simulink model "arduino_stepper"  (R2014a)
settings: Solver=FixedStepDiscrete  SolverMode=SingleTasking  StartTime=0.0  StopTime=inf  FixedStep=0.010  RelTol=1e-3
libraries: arduinolib x5
settings Model: SimulationMode=external  ExtModeTrigDuration=2  Creator=hbosch  LastModifiedBy=hbosch
settings DataIOCC: LimitDataPoints=off  SaveOutput=off  SignalLogging=off  DSMLogging=off  SaveTime=off
settings OptimizationCC: InlineParams=on  StateBitsets=on  DataBitsets=on  OptimizeModelRefInitCode=on  LifeSpan=1
settings DebuggingCC: SignalInfNanChecking=error  SignalRangeChecking=error  ReadBeforeWriteMsg=EnableAllAsError  WriteAfterWriteMsg=EnableAllAsError  WriteAfterReadMsg=EnableAllAsError  AlgebraicLoopMsg=error  ArtificialAlgebraicLoopMsg=error  SaveWithDisabledLinksMsg=error  SaveWithParameterizedLinksMsg=error  UnderspecifiedInitializationDetection=Classic  MergeDetectMultiDrivingBlocksExec=error  CheckExecutionContextPreStartOutputMsg=on  CheckExecutionContextRuntimeOutputMsg=on  BlockPriorityViolationMsg=error  TimeAdjustmentMsg=warning  SolverPrmCheckMsg=none  InheritedTsInSrcMsg=error  DiscreteInheritContinuousMsg=error  SigSpecEnsureSampleTimeMsg=error  CheckMatrixSingularityMsg=error  IntegerOverflowMsg=error  ParameterUnderflowMsg=error  ParameterPrecisionLossMsg=error  ParameterTunabilityLossMsg=error  UnderSpecifiedDataTypeMsg=error  UnnecessaryDatatypeConvMsg=warning  VectorMatrixConversionMsg=error  SignalLabelMismatchMsg=error  UnconnectedInputMsg=error  UnconnectedOutputMsg=error  UnconnectedLineMsg=error  SFcnCompatibilityMsg=error  UniqueDataStoreMsg=error  BusObjectLabelMismatch=error  RootOutportRequireBusObject=error  AssertControl=DisableAll  ModelReferenceIOMsg=error  ModelReferenceIOMismatchMessage=error  ModelReferenceCSMismatchMessage=error  UnknownTsInhSupMsg=error  ModelReferenceDataLoggingMessage=error  StateNameClashWarn=warning
settings HardwareCC: ProdBitPerInt=16  ProdBitPerPointer=8  ProdIntDivRoundTo=Zero  ProdEndianess=LittleEndian  ProdWordSize=8  ProdHWDeviceType=Atmel->AVR
settings RTWCC: SystemTargetFile=realtime.tlc  GenerateMakefile=off  TemplateMakefile=realtime.tmf  Description=Run on Target Hardware  RTWVerbose=off  ProcessScript=realtime_make_rtw_hook
settings CodeAppCC: MangleLength=10
settings STFCustomTargetCC: TargetLibSuffix=.a  GenerateSampleERTMain=on  ConcurrentExecutionCompliant=off  GeneratePreprocessorConditionals=Use local settings  ERTCustomFileBanners=on  SupportNonInlinedSFcns=off  SupportVariableSizeSignals=on  MATLABClassNameForMDSCustomization=Simulink.SoftwareTarget.ERTCustomization  GRTInterface=off  SystemTargetFile=realtime.tlc
settings ERTTargetCC: CombineOutputUpdateFcns=off  SupportContinuousTime=on  SupportVariableSizeSignals=on  ExtModeTransport=3  ExtModeMexFile=ext_serial_win32_comm  ExtModeMexArgs=0 1 9600  ERTSrcFileBannerTemplate=realtime_code_template.cgt  ERTHdrFileBannerTemplate=realtime_code_template.cgt  ERTDataSrcFileTemplate=realtime_code_template.cgt  ERTDataHdrFileTemplate=realtime_code_template.cgt  ERTCustomFileTemplate=realtime_file_process.tlc

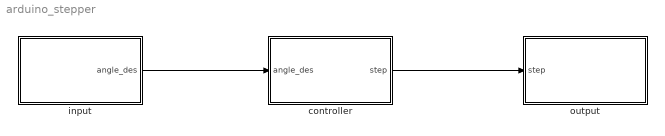
== system arduino_stepper ==
  controller : Subsystem
  input : Subsystem
  output : Subsystem
  wires:
  input/1(angle_des) -> controller/1(angle_des)
  controller/1(step) -> output/1(step)

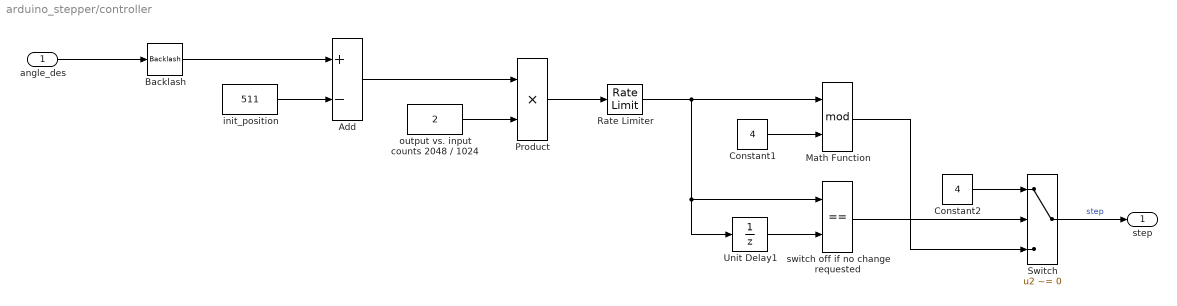
== system arduino_stepper/controller ==
  angle_des : Inport
  Add : Sum  Inputs=+-  InputSameDT=on
  Backlash : Backlash  BacklashWidth=6  InitialOutput=511
  Constant1 : Constant  Value=4  OutDataTypeStr=int16
  Constant2 : Constant  Value=4  OutDataTypeStr=int16
  Math Function : Math  Operator=mod  SaturateOnIntegerOverflow=on
  Product : Product  OutDataTypeStr=int16  RndMeth=Zero  InputSameDT=on
  Rate Limiter : RateLimiter  RisingSlewLimit=100  FallingSlewLimit=-100  SampleTimeMode=inherited
  Switch : Switch  Criteria=u2 ~= 0  InputSameDT=on
  Unit Delay1 : UnitDelay  SampleTime=-1
  init_position : Constant  Value=511  OutDataTypeStr=int16
  output vs. input counts 2048 / 1024 : Constant  Value=2  OutDataTypeStr=int16
  switch off if no change requested : RelationalOperator  Operator===  OutDataTypeStr=boolean  InputSameDT=on
  step : Outport
  wires:
  angle_des/1 -> Backlash/1
  init_position/1 -> Add/2
  Add/1 -> Product/1
  output vs. input counts 2048 / 1024/1 -> Product/2
  Product/1 -> Rate Limiter/1
  Constant1/1 -> Math Function/2
  Rate Limiter/1 -> switch off if no change requested/1, Unit Delay1/1, Math Function/1
  Backlash/1 -> Add/1
  Switch/1 -> step/1  "step"
  Constant2/1 -> Switch/1
  switch off if no change requested/1 -> Switch/2
  Math Function/1 -> Switch/3
  Unit Delay1/1 -> switch off if no change requested/2

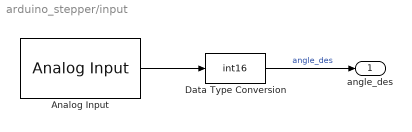
== system arduino_stepper/input ==
  Analog Input : arduinolib/Analog Input  pinNumber=0  sampleTime=0.010
  Data Type Conversion : DataTypeConversion  OutDataTypeStr=int16
  angle_des : Outport
  wires:
  Analog Input/1 -> Data Type Conversion/1
  Data Type Conversion/1 -> angle_des/1  "angle_des"

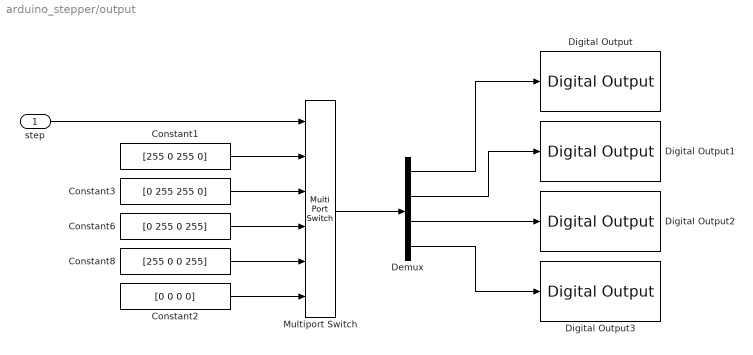
== system arduino_stepper/output ==
  step : Inport
  Constant1 : Constant  Value=[255 0 255 0]  OutDataTypeStr=uint8
  Constant2 : Constant  Value=[0 0 0 0]  OutDataTypeStr=uint8
  Constant3 : Constant  Value=[0 255 255 0]  OutDataTypeStr=uint8
  Constant6 : Constant  Value=[0 255 0 255]  OutDataTypeStr=uint8
  Constant8 : Constant  Value=[255 0 0 255]  OutDataTypeStr=uint8
  Demux : Demux
  Digital Output : arduinolib/Digital Output  pinNumber=2
  Digital Output1 : arduinolib/Digital Output  pinNumber=3
  Digital Output2 : arduinolib/Digital Output  pinNumber=4
  Digital Output3 : arduinolib/Digital Output  pinNumber=5
  Multiport Switch : MultiPortSwitch  DataPortOrder=Zero-based contiguous  Inputs=4  DataPortForDefault=Additional data port  DiagnosticForDefault=None  InputSameDT=on
  wires:
  Demux/1 -> Digital Output/1
  Demux/2 -> Digital Output1/1
  Demux/3 -> Digital Output2/1
  Demux/4 -> Digital Output3/1
  Constant1/1 -> Multiport Switch/2
  Multiport Switch/1 -> Demux/1
  step/1 -> Multiport Switch/1
  Constant3/1 -> Multiport Switch/3
  Constant6/1 -> Multiport Switch/4
  Constant8/1 -> Multiport Switch/5
  Constant2/1 -> Multiport Switch/6
